simulink model "combinedFC_NicholasSeecharan"  (R2025b)
settings: Solver=VariableStepAuto  StartTime=0.0  StopTime=10.0  RelTol=1e-3

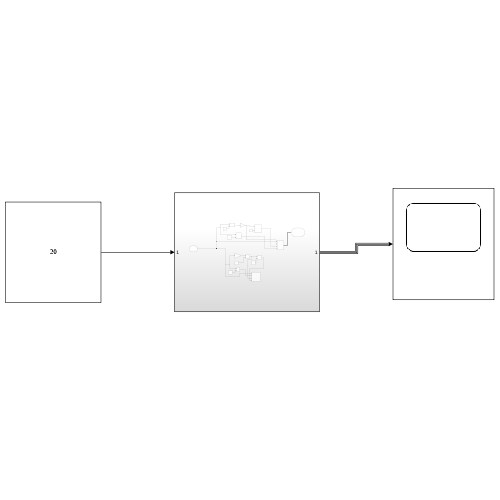
[thumbnail: Simulink's stored preview of the top-level diagram]
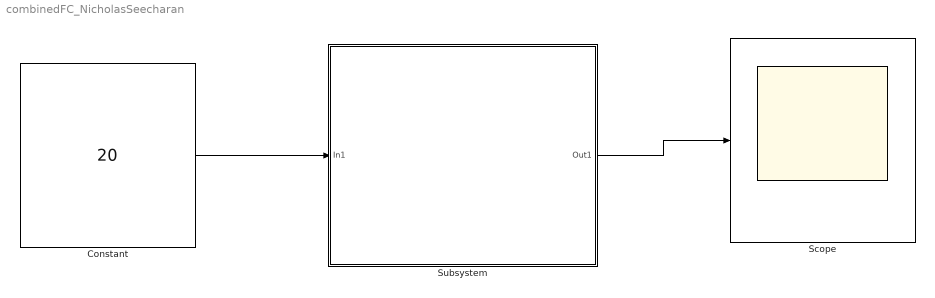
== system combinedFC_NicholasSeecharan ==
  Constant : Constant  Value=20
  Scope : Scope
      settings: ActiveDisplayYMinimum=-67.458749999999981  ActiveDisplayYMaximum=540.46208333333334
  Subsystem : Subsystem
  wires:
  Constant/1 -> Subsystem/1(In1)
  Subsystem/1(Out1) -> Scope/1

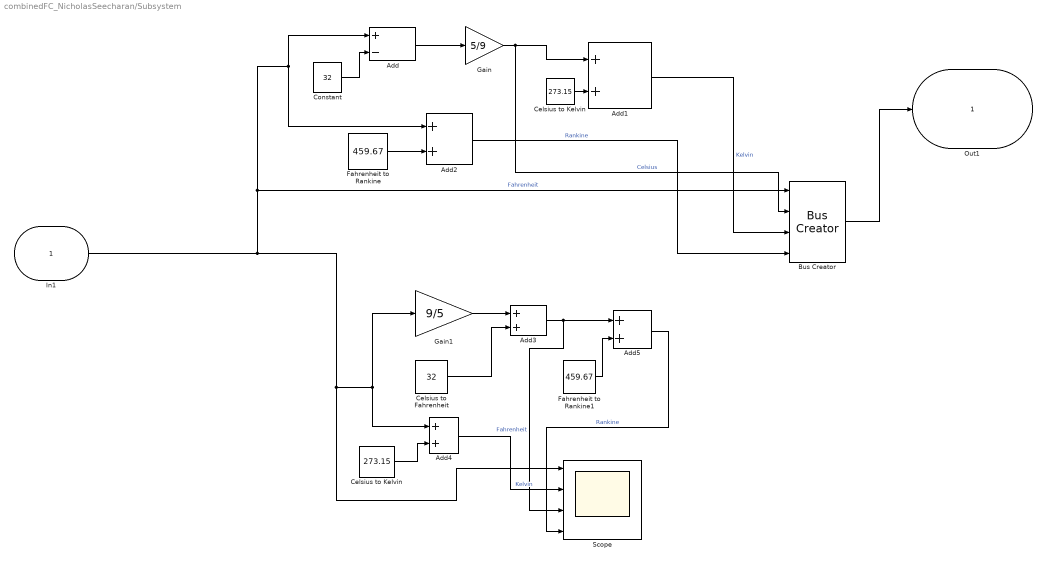
== system combinedFC_NicholasSeecharan/Subsystem ==
  In1 : Inport
  Add : Sum  Inputs=+-
  Add{1..5} (5 alike) : Sum
  Bus Creator : BusCreator  Inputs=4
  Celsius to Fahrenheit : Constant  Value=32
  Celsius to Kelvin : Constant  Value=273.15
  "Celsius to Kelvin " : Constant  Value=273.15
  Constant : Constant  Value=32
  Fahrenheit to Rankine : Constant  Value=459.67
  Fahrenheit to Rankine1 : Constant  Value=459.67
  Gain : Gain  Gain=5/9
  Gain1 : Gain  Gain=9/5
  Scope : Scope  NumInputPorts=4
      settings: SampleTime=10  Title=Celsius Converter  ActiveDisplayYMinimum=-16.458749999999995  ActiveDisplayYMaximum=648.12875000000008  YLabel=Celsius
  Out1 : Outport
  wires:
  Celsius to Kelvin/1 -> Add1/2
  Add1/1 -> Bus Creator/3  "Kelvin"
  Gain/1 -> Bus Creator/2, Add1/1  "Celsius"
  Add2/1 -> Bus Creator/4  "Rankine"
  Add/1 -> Gain/1
  Constant/1 -> Add/2
  Fahrenheit to Rankine/1 -> Add2/2
  "Celsius to Kelvin "/1 -> Add4/2
  Celsius to Fahrenheit/1 -> Add3/2
  Add5/1 -> Scope/4  "Rankine"
  Add3/1 -> Scope/3, Add5/1  "Fahrenheit"
  In1/1 -> Scope/1, Gain1/1, Add4/1, Bus Creator/1, Add2/1, Add/1  "Fahrenheit"
  Fahrenheit to Rankine1/1 -> Add5/2
  Gain1/1 -> Add3/1
  Add4/1 -> Scope/2  "Kelvin"
  Bus Creator/1 -> Out1/1
